simulink model "teste_espalhamento"  (R2014a)
settings: Solver=ode3  StartTime=0.0  StopTime=10.0  RelTol=1e-3
libraries: dspsigops x1
settings Model: Creator=andre  LastModifiedBy=andre

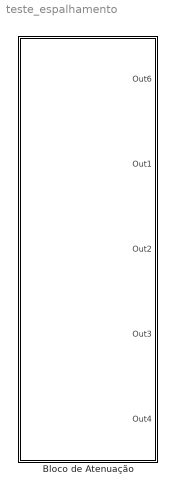
== system teste_espalhamento ==
  Bloco de Atenuação : Subsystem

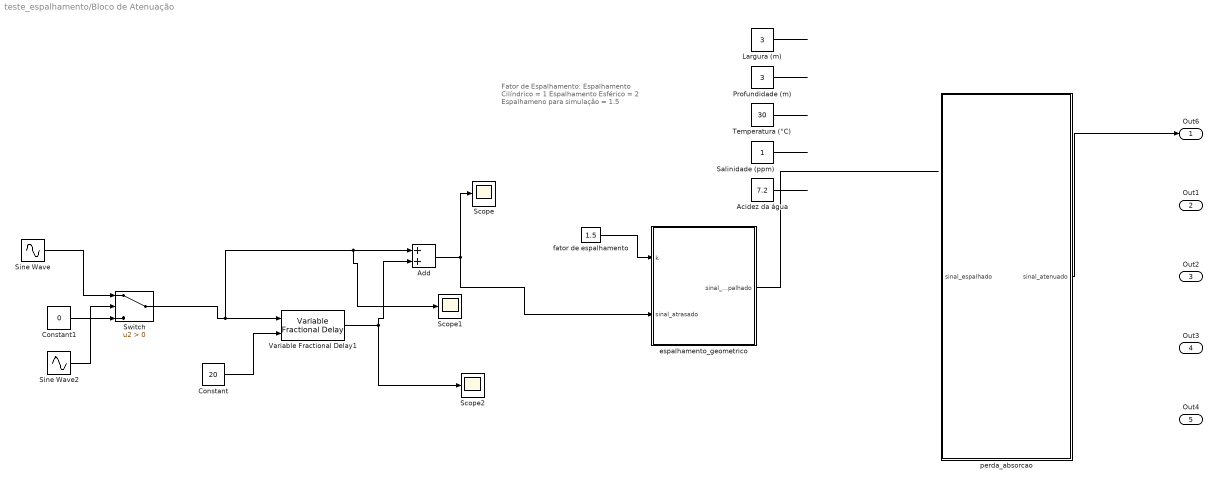
== system teste_espalhamento/Bloco de Atenuação ==
  note: Fator de Espalhamento:
      |
      | Espalhamento Cilíndrico = 1
      | Espalhamento Esférico = 2
      | Espalhameno para simulação = 1.5
  Acidez da água : Constant  Value=7.2
  Add : Sum
  Constant : Constant  Value=20  SampleTime=0
  Constant1 : Constant  Value=0
  Largura (m) : Constant  Value=3
  Profundidade (m) : Constant  Value=3
  Salinidade (ppm) : Constant
  Scope : Scope
      settings: SampleTime=1000
  Scope1 : Scope
      settings: SampleTime=1000
  Scope2 : Scope
      settings: SaveName=ScopeData2  SampleTime=1000
  Sine Wave : Sin  SineType=Sample based  Amplitude=3  Frequency=100  Samples=20  SampleTime=1/20000
  Sine Wave2 : Sin  SampleTime=1/20000
  Switch : Switch  Criteria=u2 > Threshold
  Temperatura (°C) : Constant  Value=30
  Variable Fractional Delay1 : dspsigops/Variable Fractional Delay  mode=OBSOLETE  modeActive=Linear  dmax=10000  InputProcessing=Columns as channels (frame based)  L=4  FarrowL=4  R=10  alpha=1  ic=0  fallbackFIR=Clip to the minimum value necessary for centered kernel  fallbackFarrow=Clip to the minimum value necessary for centered kernel  noDFT=off  roundingMode=Zero  overflowMode=off
  espalhamento_geometrico : MATLAB Function  TreatAsAtomicUnit=on
  fator de espalhamento : Constant  Value=1.5
  perda_absorcao : MATLAB Function  TreatAsAtomicUnit=on
  Out6 : Outport
  Out1 : Outport  Port=2
  Out2 : Outport  Port=3
  Out3 : Outport  Port=4
  Out4 : Outport  Port=5
  wires:
  espalhamento_geometrico/1(sinal_espalhado) -> ?
  fator de espalhamento/1 -> espalhamento_geometrico/1(k)
  perda_absorcao/1(sinal_atenuado) -> Out6/1
  ? -> Out1/1
  ? -> Out2/1
  ? -> Out3/1
  ? -> Out4/1
  Constant/1 -> Variable Fractional Delay1/2
  Variable Fractional Delay1/1 -> Add/2, Scope2/1
  Add/1 -> espalhamento_geometrico/2(sinal_atrasado), Scope/1
  Sine Wave/1 -> Switch/1
  Sine Wave2/1 -> Switch/2
  Constant1/1 -> Switch/3
  Switch/1 -> Scope1/1, Add/1, Variable Fractional Delay1/1
  Largura (m)/1 -> ?
  Profundidade (m)/1 -> ?
  Temperatura (°C)/1 -> ?
  Salinidade (ppm)/1 -> ?
  Acidez da água/1 -> ?

== matlab function teste_espalhamento/Bloco de Atenuação/perda_absorcao ==
  data: sinal_espalhado input; sinal_atenuado output
function sinal_atenuado   = perda_absorcao(sinal_espalhado)
% Calcular o coeficeinte de absorção (a)
% Calcular a perda por absorção

% Parâmetros Ambientais
T = 32;      % Temperatura da água
S = 1;       % Salinidade da água
pH = 7.2;      % Acidez da água

% Parâmetro da Geometria do Aquário
D = 3;          % Profundidade

frequencia = 19670;

%Valores dos parâmetros Ácido Bórico(f1) e Sulfato de Magnésio(f2)
f1 = 0.78 * sqrt(S/35) * (exp(T/26));
f2 = 42 * (exp(T/17));

%--------------------------------------------------------------------------
% Coeficiente de Absorção (a) 
% Depende diretamente da frequencia do sinal e das frequências (f1) e (f2)
%--------------------------------------------------------------------------
a = ((0.106 * (f1 * frequencia^2) * exp((pH - 8)/0.56)) / (f1^2 + frequencia^2)) +...
    ((0.52 * (1 + (T/43)) * (S/45) * (f2 * frequencia^2) *...
    exp(-(D/6))) / (f2^2 + frequencia^2)) + (0.00049 * (frequencia^2) * (exp(-(T/27 + D/17))));

%--------------------------------------------------------------------------
% Perda_absorção = 10log(a)*r (dB)
% Esse coeficiente varia linerarmente com a faixa r em quilômetros para um
% dado valor de frequência
%--------------------------------------------------------------------------
atenuacao = -10*log10(a)*caminho;

%-------------------------------------------------------------------------
% Equação para o espalhamento do sinal utilizando a razao normal de ganho
% em que G=(Pout/Pin)<1
% in = sinal_espalhado*10^(atenuacao/10) 
%-------------------------------------------------------------------------

sinal_atenuado = sinal_espalhado.*(10^(atenuacao/10));
%-------------------------------------------------------------------------
%Soma dos sinais atenuados representando o sinal atenuado total
%-------------------------------------------------------------------------

== matlab function teste_espalhamento/Bloco de Atenuação/espalhamento_geometrico ==
  data: k input; sinal_atrasado input; sinal_espalhado output
function sinal_espalhado  = espalhamento_geometrico(k,sinal_atrasado)
%a perda por espalhamento geométrico é calculado a partir da equação 
%perda_espalhamento = k * 10log(r); equação da dissertação
%k = fator de espalhamento
%caminhos = distância em metros que o sinal percorre ao longo da propagação

caminho = 10;
%-------------------------------------------------------------------------
%Equação para cálculo da perda por espalhamento geométrico (Spreading Loss)
%-------------------------------------------------------------------------
espalhamento = -k * 10*log10(caminho);

%-------------------------------------------------------------------------
% Equação para o espalhamento do sinal utilizando a razao normal de ganho
% em que G=(Pout/Pin)<1
% in = sinal_atrasado*10^(espelhamento/10)
%-------------------------------------------------------------------------
sinal_espalhado = sinal_atrasado.*(10^(espalhamento/10));
